simulink model "OMAP"  (R2018b)
settings: Solver=FixedStepDiscrete  StartTime=0.0  StopTime=10.0  FixedStep=0.01  RelTol=1e-3
values from neighbouring files (symbols this model uses):
  Clb_ICADirect_LaneDisp_StateFive = Simulink.Parameter    [omap_ver_442.m]
  Clb_ICADirect_LaneDisp_StateFour = Simulink.Parameter    [omap_ver_442.m]
  Clb_ICADirect_LaneDisp_StateOne = Simulink.Parameter    [omap_ver_442.m]
  Clb_ICADirect_LaneDisp_StateThree = Simulink.Parameter    [omap_ver_442.m]
  Clb_ICADirect_LaneDisp_StateTwo = Simulink.Parameter    [omap_ver_442.m]
  Clb_ICADirect_LaneDisp_StateZero = Simulink.Parameter    [omap_ver_442.m]
  Clb_ICADirect_LaneDispSW = Simulink.Parameter    [omap_ver_442.m]
  Clb_ICADirect_TrnLghtsCom_Switch = Simulink.Parameter    [omap_ver_442.m]
  Clb_ICADirect_TrnLghtsCom_Value = Simulink.Parameter    [omap_ver_442.m]
  Clb_ICADirect_TrnLghtsCrtl_Inhb = Simulink.Parameter    [omap_ver_442.m]
  OMAP_ACCAEB_EMSESC_Decel = Simulink.Parameter    [omap_ver_442.m]
  OMAP_ACCFCW_IC_Decel = Simulink.Parameter    [omap_ver_442.m]
  OMAP_clb_ACC_RVVReqType = Simulink.Parameter    [omap_ver_442.m]
  OMAP_clb_ACC_RVVReqType_Switch = Simulink.Parameter    [omap_ver_442.m]
  OMAP_clb_ACCHeadwayDisplay = Simulink.Parameter    [omap_ver_442.m]
  OMAP_clb_ACCHeadwayDisplay_Switch = Simulink.Parameter    [omap_ver_442.m]
  OMAP_clb_ACCHeadwayIcon = Simulink.Parameter    [omap_ver_442.m]
  OMAP_clb_ACCHeadwayIcon_Switch = Simulink.Parameter    [omap_ver_442.m]
  OMAP_clb_ACCMessagePrompt = Simulink.Parameter    [omap_ver_442.m]
  OMAP_clb_ACCMessagePrompt_Switch = Simulink.Parameter    [omap_ver_442.m]
  OMAP_clb_ACCRequestEPB = Simulink.Parameter    [omap_ver_442.m]
  OMAP_clb_ACCRequestEPB_Switch = Simulink.Parameter    [omap_ver_442.m]
  OMAP_clb_ACCSetSpeed = Simulink.Parameter    [omap_ver_442.m]
  OMAP_clb_ACCSetSpeed_Switch = Simulink.Parameter    [omap_ver_442.m]
  OMAP_clb_ACCSetSpeedDis = Simulink.Parameter    [omap_ver_442.m]
  OMAP_clb_ACCSetSpeedDis_Switch = Simulink.Parameter    [omap_ver_442.m]
  OMAP_clb_ACCState = Simulink.Parameter    [omap_ver_442.m]
  OMAP_clb_ACCState_Switch = Simulink.Parameter    [omap_ver_442.m]
  OMAP_clb_ACCStatusIconDis = Simulink.Parameter    [omap_ver_442.m]
  OMAP_clb_ACCStatusIconDis_Switch = Simulink.Parameter    [omap_ver_442.m]
  OMAP_clb_ACCTorqueReq = Simulink.Parameter    [omap_ver_442.m]
  OMAP_clb_ACCTorqueReq_Switch = Simulink.Parameter    [omap_ver_442.m]
  OMAP_clb_ADAS_State = Simulink.Parameter    [omap_ver_442.m]
  OMAP_clb_ADAS_State_Switch = Simulink.Parameter    [omap_ver_442.m]
  OMAP_clb_AEBAlertReq = Simulink.Parameter    [omap_ver_442.m]
  OMAP_clb_AEBAlertReq_Switch = Simulink.Parameter    [omap_ver_442.m]
  OMAP_clb_AEBBrakingProg = Simulink.Parameter    [omap_ver_442.m]
  OMAP_clb_AEBBrakingProg_Switch = Simulink.Parameter    [omap_ver_442.m]
  OMAP_clb_AEBFaultStatus = Simulink.Parameter    [omap_ver_442.m]
  OMAP_clb_AEBFaultStatus_Switch = Simulink.Parameter    [omap_ver_442.m]
  OMAP_clb_AEBMassageDisp = Simulink.Parameter    [omap_ver_442.m]
  OMAP_clb_AEBMassageDisp_Switch = Simulink.Parameter    [omap_ver_442.m]
  OMAP_clb_AEBState = Simulink.Parameter    [omap_ver_442.m]
  OMAP_clb_AEBState_Switch = Simulink.Parameter    [omap_ver_442.m]
  OMAP_clb_AEBSwitchStatus = Simulink.Parameter    [omap_ver_442.m]
  OMAP_clb_AEBSwitchStatus_Switch = Simulink.Parameter    [omap_ver_442.m]
  OMAP_clb_BrakeRequest = Simulink.Parameter    [omap_ver_442.m]
  OMAP_clb_BrakeRequest_Switch = Simulink.Parameter    [omap_ver_442.m]
  OMAP_clb_DecelerationSet = Simulink.Parameter    [omap_ver_442.m]
  OMAP_clb_DecelerationSet_Switch = Simulink.Parameter    [omap_ver_442.m]
  OMAP_clb_DecelerationType = Simulink.Parameter    [omap_ver_442.m]
  OMAP_clb_DecelerationType_Switch = Simulink.Parameter    [omap_ver_442.m]
  OMAP_clb_DeclControlReq = Simulink.Parameter    [omap_ver_442.m]
  OMAP_clb_DeclControlReq_Switch = Simulink.Parameter    [omap_ver_442.m]
  OMAP_clb_DownorUpGearMinTime = Simulink.Parameter    [omap_ver_442.m]
  OMAP_clb_DownorUpGearMinTime_Switch = Simulink.Parameter    [omap_ver_442.m]
  OMAP_clb_ELKPopupMessage = Simulink.Parameter    [omap_ver_442.m]
  OMAP_clb_ELKPopupMessage_Switch = Simulink.Parameter    [omap_ver_442.m]
  OMAP_clb_ELKSts = Simulink.Parameter    [omap_ver_442.m]
  OMAP_clb_ELKSts_Switch = Simulink.Parameter    [omap_ver_442.m]
  OMAP_clb_ESAFaultSt = Simulink.Parameter    [omap_ver_442.m]
  OMAP_clb_ESAFaultSt_Switch = Simulink.Parameter    [omap_ver_442.m]
  OMAP_clb_ESARequest = Simulink.Parameter    [omap_ver_442.m]
  OMAP_clb_ESARequest_Switch = Simulink.Parameter    [omap_ver_442.m]
  OMAP_clb_ESAState = Simulink.Parameter    [omap_ver_442.m]
  OMAP_clb_ESAState_Switch = Simulink.Parameter    [omap_ver_442.m]
  OMAP_clb_ESATorqueReq = Simulink.Parameter    [omap_ver_442.m]
  OMAP_clb_ESATorqueReq_Switch = Simulink.Parameter    [omap_ver_442.m]
  OMAP_clb_ESCDriveOff = Simulink.Parameter    [omap_ver_442.m]
  OMAP_clb_ESCDriveOff_Switch = Simulink.Parameter    [omap_ver_442.m]
  OMAP_clb_ESCHoldReq = Simulink.Parameter    [omap_ver_442.m]
  OMAP_clb_ESCHoldReq_Switch = Simulink.Parameter    [omap_ver_442.m]
  OMAP_clb_Handsoffwarning = Simulink.Parameter    [omap_ver_442.m]
  OMAP_clb_Handsoffwarning_Switch = Simulink.Parameter    [omap_ver_442.m]
  OMAP_clb_HapticAlarmReq = Simulink.Parameter    [omap_ver_442.m]
  OMAP_clb_HapticAlarmReq_Switch = Simulink.Parameter    [omap_ver_442.m]
  OMAP_clb_HMIPopupMassage = Simulink.Parameter    [omap_ver_442.m]
  OMAP_clb_HMIPopupMassage_Switch = Simulink.Parameter    [omap_ver_442.m]
  OMAP_clb_HWAActionSts = Simulink.Parameter    [omap_ver_442.m]
  OMAP_clb_HWAActionSts_Switch = Simulink.Parameter    [omap_ver_442.m]
  OMAP_clb_HWAMode = Simulink.Parameter    [omap_ver_442.m]
  OMAP_clb_HWAMode_Switch = Simulink.Parameter    [omap_ver_442.m]
  OMAP_clb_HWATurnOnIdctr = Simulink.Parameter    [omap_ver_442.m]
  OMAP_clb_HWATurnOnIdctr_Switch = Simulink.Parameter    [omap_ver_442.m]
  OMAP_clb_ICAMassageDisp = Simulink.Parameter    [omap_ver_442.m]
  OMAP_clb_ICAMassageDisp_Switch = Simulink.Parameter    [omap_ver_442.m]
  OMAP_clb_ICAStatusIcon = Simulink.Parameter    [omap_ver_442.m]
  OMAP_clb_ICAStatusIcon_Switch = Simulink.Parameter    [omap_ver_442.m]
  OMAP_clb_ISLCDriverRemind = Simulink.Parameter    [omap_ver_442.m]
  OMAP_clb_ISLCDriverRemind_Switch = Simulink.Parameter    [omap_ver_442.m]
  OMAP_clb_ISLCState = Simulink.Parameter    [omap_ver_442.m]
  OMAP_clb_ISLCState_Switch = Simulink.Parameter    [omap_ver_442.m]
  OMAP_clb_JAFaultSt = Simulink.Parameter    [omap_ver_442.m]
  OMAP_clb_JAFaultSt_Switch = Simulink.Parameter    [omap_ver_442.m]
  OMAP_clb_LCAPopupMessage = Simulink.Parameter    [omap_ver_442.m]
  OMAP_clb_LCAPopupMessage_Switch = Simulink.Parameter    [omap_ver_442.m]
  OMAP_clb_LCAStatusDisplay = Simulink.Parameter    [omap_ver_442.m]
  OMAP_clb_LCAStatusDisplay_Switch = Simulink.Parameter    [omap_ver_442.m]
  OMAP_clb_LDWStatusDisplay = Simulink.Parameter    [omap_ver_442.m]
  OMAP_clb_LDWStatusDisplay_Switch = Simulink.Parameter    [omap_ver_442.m]
  OMAP_clb_LDWWarningSt = Simulink.Parameter    [omap_ver_442.m]
  OMAP_clb_LDWWarningSt_Switch = Simulink.Parameter    [omap_ver_442.m]
  OMAP_clb_LightControlValid = Simulink.Parameter    [omap_ver_442.m]
  OMAP_clb_LightControlValid_Switch = Simulink.Parameter    [omap_ver_442.m]
  OMAP_clb_LKAActivation = Simulink.Parameter    [omap_ver_442.m]
  OMAP_clb_LKAActivation_Switch = Simulink.Parameter    [omap_ver_442.m]
  OMAP_clb_LKAAngleReq = Simulink.Parameter    [omap_ver_442.m]
  OMAP_clb_LKAAngleReq_Switch = Simulink.Parameter    [omap_ver_442.m]
  OMAP_clb_LKAMode = Simulink.Parameter    [omap_ver_442.m]
  OMAP_clb_LKAMode_Switch = Simulink.Parameter    [omap_ver_442.m]
  OMAP_clb_LKAorELK_CoolTime = Simulink.Parameter    [omap_ver_442.m]
  OMAP_clb_LKAState = Simulink.Parameter    [omap_ver_442.m]
  OMAP_clb_LKAState_Switch = Simulink.Parameter    [omap_ver_442.m]
  OMAP_clb_LKAStatusDisplay = Simulink.Parameter    [omap_ver_442.m]
  OMAP_clb_LKAStatusDisplay_Switch = Simulink.Parameter    [omap_ver_442.m]
  OMAP_clb_LKASwitchState = Simulink.Parameter    [omap_ver_442.m]
  OMAP_clb_LKASwitchState_Switch = Simulink.Parameter    [omap_ver_442.m]
  OMAP_clb_LKATorqFactReq = Simulink.Parameter    [omap_ver_442.m]
  OMAP_clb_LKATorqFactReq_Switch = Simulink.Parameter    [omap_ver_442.m]
  OMAP_clb_PrefillRequest = Simulink.Parameter    [omap_ver_442.m]
  ... (+36 more)
libraries: simulink x184, canmsglib x2
(part 11 of 14)

== system OMAP/Runnable_OMAP_10ms_sys/OMAP_Module/ACCS_Direct/ACCS_Define/Human_Machine_Interface(ACC_HMI)/Text_PopUp/ACC_Canceled ==
  In1 : Inport
  Chart : Stateflow chart  TreatAsAtomicUnit=on
  Compare To Constant1 : simulink/Logic and Bit Operations/Compare To Constant  relop===  const=2  OutDataTypeStr=boolean
  Compare To Constant2 : simulink/Logic and Bit Operations/Compare To Constant  relop===  const=3  OutDataTypeStr=boolean
  Compare To Constant23 : simulink/Logic and Bit Operations/Compare To Constant  relop===  const=4  OutDataTypeStr=boolean
  Compare To Constant3 : simulink/Logic and Bit Operations/Compare To Constant  relop===  const=7  OutDataTypeStr=boolean
  Compare To Constant4 : simulink/Logic and Bit Operations/Compare To Constant  relop===  const=6  OutDataTypeStr=boolean
  Compare To Constant5 : simulink/Logic and Bit Operations/Compare To Constant  relop===  const=2  OutDataTypeStr=boolean
  Compare To Constant6 : simulink/Logic and Bit Operations/Compare To Constant  relop===  const=3  OutDataTypeStr=boolean
  Compare To Constant7 : simulink/Logic and Bit Operations/Compare To Constant  relop===  const=5  OutDataTypeStr=boolean
  Logical Operator1 : Logic  Operator=OR  Inputs=3  AllPortsSameDT=off  OutDataTypeStr=boolean
  Logical Operator16 : Logic  AllPortsSameDT=off  OutDataTypeStr=boolean
  Logical Operator2 : Logic  Operator=OR  AllPortsSameDT=off  OutDataTypeStr=boolean
  Logical Operator3 : Logic  Operator=OR  AllPortsSameDT=off  OutDataTypeStr=boolean
  Logical Operator4 : Logic  AllPortsSameDT=off  OutDataTypeStr=boolean
  Logical Operator5 : Logic  Operator=OR  AllPortsSameDT=off  OutDataTypeStr=boolean
  Unit Delay1 : UnitDelay  SampleTime=-1
  Unit Delay5 : UnitDelay  SampleTime=-1
  Out1 : Outport
  wires:
  Compare To Constant1/1 -> Logical Operator1/1
  Compare To Constant23/1 -> Logical Operator16/1
  Logical Operator16/1 -> Logical Operator2/1
  Chart/1(Value) -> Out1/1
  Unit Delay5/1 -> Compare To Constant23/1
  Compare To Constant2/1 -> Logical Operator1/2
  Compare To Constant3/1 -> Logical Operator1/3
  Logical Operator1/1 -> Logical Operator16/2
  Compare To Constant5/1 -> Logical Operator3/1
  Compare To Constant7/1 -> Logical Operator5/1
  In1/1 -> Compare To Constant6/1, Compare To Constant5/1, Unit Delay1/1, Compare To Constant3/1, Compare To Constant2/1, Compare To Constant1/1, Unit Delay5/1
  Unit Delay1/1 -> Compare To Constant4/1, Compare To Constant7/1
  Compare To Constant6/1 -> Logical Operator3/2
  Logical Operator3/1 -> Logical Operator4/2
  Logical Operator4/1 -> Logical Operator2/2
  Logical Operator2/1 -> Chart/1(data)
  Compare To Constant4/1 -> Logical Operator5/2
  Logical Operator5/1 -> Logical Operator4/1

== system OMAP/Runnable_OMAP_10ms_sys/OMAP_Module/ACCS_Direct/ACCS_Define/Human_Machine_Interface(ACC_HMI)/Text_PopUp/ACC_Fault ==
  In1 : Inport
  Chart : Stateflow chart  TreatAsAtomicUnit=on
  Compare To Constant1 : simulink/Logic and Bit Operations/Compare To Constant  relop=~=  const=15  OutDataTypeStr=boolean
  Compare To Constant15 : simulink/Logic and Bit Operations/Compare To Constant  relop===  const=15  OutDataTypeStr=boolean
  Logical Operator : Logic  AllPortsSameDT=off  OutDataTypeStr=boolean
  Unit Delay : UnitDelay  SampleTime=-1
  Out1 : Outport
  wires:
  Logical Operator/1 -> Chart/1(data)
  In1/1 -> Compare To Constant15/1, Unit Delay/1
  Compare To Constant1/1 -> Logical Operator/1
  Compare To Constant15/1 -> Logical Operator/2
  Unit Delay/1 -> Compare To Constant1/1
  Chart/1(Value) -> Out1/1

== system OMAP/Runnable_OMAP_10ms_sys/OMAP_Module/ACCS_Direct/ACCS_Define/Human_Machine_Interface(ACC_HMI)/Text_PopUp/ACC_OFF ==
  In1 : Inport
  In2 : Inport  Port=2
  Chart : Stateflow chart  TreatAsAtomicUnit=on
  Compare To Constant1 : simulink/Logic and Bit Operations/Compare To Constant  relop===  const=1  OutDataTypeStr=boolean
  Compare To Constant10 : simulink/Logic and Bit Operations/Compare To Constant  relop===  const=8  OutDataTypeStr=boolean
  Compare To Constant2 : simulink/Logic and Bit Operations/Compare To Constant  relop=~=  const=0  OutDataTypeStr=boolean
  Compare To Constant3 : simulink/Logic and Bit Operations/Compare To Constant  relop=~=  const=15  OutDataTypeStr=boolean
  Compare To Constant4 : simulink/Logic and Bit Operations/Compare To Constant  relop=~=  const=1  OutDataTypeStr=boolean
  Compare To Constant5 : simulink/Logic and Bit Operations/Compare To Constant  relop=~=  const=8  OutDataTypeStr=boolean
  Compare To Constant6 : simulink/Logic and Bit Operations/Compare To Constant  relop===  const=0  OutDataTypeStr=boolean
  Compare To Constant7 : simulink/Logic and Bit Operations/Compare To Constant  relop===  const=1  OutDataTypeStr=boolean
  Compare To Constant8 : simulink/Logic and Bit Operations/Compare To Constant  relop===  const=4  OutDataTypeStr=boolean
  Logical Operator1 : Logic  Inputs=4  AllPortsSameDT=off  OutDataTypeStr=boolean
  Logical Operator2 : Logic  AllPortsSameDT=off  OutDataTypeStr=boolean
  Logical Operator3 : Logic  AllPortsSameDT=off  OutDataTypeStr=boolean
  Logical Operator4 : Logic  Operator=OR  AllPortsSameDT=off  OutDataTypeStr=boolean
  Logical Operator5 : Logic  AllPortsSameDT=off  OutDataTypeStr=boolean
  Unit Delay1 : UnitDelay  SampleTime=-1
  Unit Delay2 : UnitDelay  SampleTime=-1
  Unit Delay6 : UnitDelay  SampleTime=-1
  Out1 : Outport
  wires:
  Unit Delay6/1 -> Compare To Constant8/1
  Logical Operator3/1 -> Logical Operator4/1
  Compare To Constant10/1 -> Logical Operator3/2
  Compare To Constant8/1 -> Logical Operator3/1
  Chart/1(Value) -> Out1/1
  Unit Delay1/1 -> Compare To Constant5/1, Compare To Constant4/1, Compare To Constant3/1, Compare To Constant2/1
  Compare To Constant1/1 -> Logical Operator2/2
  Compare To Constant2/1 -> Logical Operator1/1
  In1/1 -> Unit Delay1/1, Compare To Constant1/1, Compare To Constant10/1, Unit Delay6/1
  Compare To Constant3/1 -> Logical Operator1/2
  Compare To Constant4/1 -> Logical Operator1/3
  Compare To Constant5/1 -> Logical Operator1/4
  Logical Operator1/1 -> Logical Operator2/1
  Logical Operator2/1 -> Logical Operator4/2
  Logical Operator4/1 -> Chart/1(data)
  In2/1 -> Unit Delay2/1, Compare To Constant6/1
  Compare To Constant7/1 -> Logical Operator5/1
  Compare To Constant6/1 -> Logical Operator5/2
  Unit Delay2/1 -> Compare To Constant7/1
  Logical Operator5/1 -> Chart/2(data1)

== system OMAP/Runnable_OMAP_10ms_sys/OMAP_Module/ACCS_Direct/ACCS_Define/Human_Machine_Interface(ACC_HMI)/Text_PopUp/ACC_ON ==
  In1 : Inport
  In2 : Inport  Port=2
  ACCICA_Flag : Inport  Port=3
  Chart : Stateflow chart  TreatAsAtomicUnit=on
  Compare To Constant{1..2,6,9} (4 alike) : simulink/Logic and Bit Operations/Compare To Constant  relop===  const=1  OutDataTypeStr=boolean
  Compare To Constant10 : simulink/Logic and Bit Operations/Compare To Constant  relop=~=  const=1  OutDataTypeStr=boolean
  Compare To Constant11 : simulink/Logic and Bit Operations/Compare To Constant  relop=~=  const=15  OutDataTypeStr=boolean
  Compare To Constant14 : simulink/Logic and Bit Operations/Compare To Constant  relop===  const=3  OutDataTypeStr=boolean
  Compare To Constant3 : simulink/Logic and Bit Operations/Compare To Constant  relop===  const=2  OutDataTypeStr=boolean
  Compare To Constant4 : simulink/Logic and Bit Operations/Compare To Constant  relop=~=  const=1  OutDataTypeStr=boolean
  Compare To Constant5 : simulink/Logic and Bit Operations/Compare To Constant  relop=~=  const=0  OutDataTypeStr=boolean
  Compare To Constant7 : simulink/Logic and Bit Operations/Compare To Constant  relop===  const=0  OutDataTypeStr=boolean
  Compare To Constant8 : simulink/Logic and Bit Operations/Compare To Constant  relop===  const=0  OutDataTypeStr=boolean
  Logical Operator : Logic  Inputs=3  AllPortsSameDT=off  OutDataTypeStr=boolean
  Logical Operator1 : Logic  AllPortsSameDT=off  OutDataTypeStr=boolean
  Logical Operator2 : Logic  AllPortsSameDT=off  OutDataTypeStr=boolean
  Logical Operator3 : Logic  AllPortsSameDT=off  OutDataTypeStr=boolean
  Logical Operator4 : Logic  Operator=OR  AllPortsSameDT=off  OutDataTypeStr=boolean
  Logical Operator5 : Logic  Inputs=3  AllPortsSameDT=off  OutDataTypeStr=boolean
  Logical Operator9 : Logic  Operator=OR  AllPortsSameDT=off  OutDataTypeStr=boolean
  Unit Delay : UnitDelay  SampleTime=-1
  Unit Delay1 : UnitDelay  SampleTime=-1
  Unit Delay2 : UnitDelay  SampleTime=-1
  Out1 : Outport
  wires:
  Compare To Constant14/1 -> Logical Operator9/2
  Compare To Constant1/1 -> Logical Operator/1
  Logical Operator/1 -> Chart/1(data)
  Logical Operator9/1 -> Logical Operator/2
  Unit Delay/1 -> Compare To Constant1/1
  Compare To Constant3/1 -> Logical Operator9/1
  Chart/1(Value) -> Out1/1
  In2/1 -> Compare To Constant4/1, Unit Delay1/1
  Unit Delay1/1 -> Compare To Constant2/1
  Compare To Constant2/1 -> Logical Operator1/1
  Compare To Constant4/1 -> Logical Operator1/2
  Logical Operator4/1 -> Chart/2(data1)
  In1/1 -> Compare To Constant11/1, Compare To Constant10/1, Compare To Constant5/1, Compare To Constant14/1, Compare To Constant3/1, Unit Delay/1
  Logical Operator5/1 -> Logical Operator2/2
  ACCICA_Flag/1 -> Compare To Constant8/1, Compare To Constant9/1, Compare To Constant7/1, Unit Delay2/1
  Unit Delay2/1 -> Compare To Constant6/1
  Compare To Constant6/1 -> Logical Operator3/1
  Compare To Constant7/1 -> Logical Operator3/2
  Logical Operator3/1 -> Logical Operator2/1
  Logical Operator2/1 -> Chart/3(data2)
  Compare To Constant8/1 -> Logical Operator/3
  Logical Operator1/1 -> Logical Operator4/2
  Compare To Constant9/1 -> Logical Operator4/1
  Compare To Constant5/1 -> Logical Operator5/1
  Compare To Constant10/1 -> Logical Operator5/2
  Compare To Constant11/1 -> Logical Operator5/3

== system OMAP/Runnable_OMAP_10ms_sys/OMAP_Module/ACCS_Direct/ACCS_Define/Human_Machine_Interface(ACC_HMI)/Text_PopUp/ACC_go_request ==
  In1 : Inport
  Compare To Constant1 : simulink/Logic and Bit Operations/Compare To Constant  relop===  const=1  OutDataTypeStr=boolean
  <GoRequest> : Outport
  wires:
  In1/1 -> Compare To Constant1/1
  Compare To Constant1/1 -> <GoRequest>/1

== system OMAP/Runnable_OMAP_10ms_sys/OMAP_Module/ACCS_Direct/ACCS_Define/Human_Machine_Interface(ACC_HMI)/Text_PopUp/Please_Take_Over_the_Car ==
  In1 : Inport
  Chart1 : Stateflow chart  TreatAsAtomicUnit=on
  Compare To Constant1 : simulink/Logic and Bit Operations/Compare To Constant  relop===  const=6  OutDataTypeStr=boolean
  Compare To Constant18 : simulink/Logic and Bit Operations/Compare To Constant  relop===  const=6  OutDataTypeStr=boolean
  Compare To Constant19 : simulink/Logic and Bit Operations/Compare To Constant  relop===  const=4  OutDataTypeStr=boolean
  Compare To Constant2 : simulink/Logic and Bit Operations/Compare To Constant  relop=~=  const=6  OutDataTypeStr=boolean
  Logical Operator1 : Logic  AllPortsSameDT=off  OutDataTypeStr=boolean
  Logical Operator7 : Logic  AllPortsSameDT=off  OutDataTypeStr=boolean
  Unit Delay1 : UnitDelay  SampleTime=-1
  Unit Delay2 : UnitDelay  SampleTime=-1
  Out1 : Outport
  wires:
  Logical Operator7/1 -> Chart1/1(IN)
  Compare To Constant18/1 -> Logical Operator7/2
  Unit Delay2/1 -> Compare To Constant19/1
  Compare To Constant19/1 -> Logical Operator7/1
  Chart1/1(Value) -> Out1/1
  Unit Delay1/1 -> Compare To Constant1/1
  Compare To Constant1/1 -> Logical Operator1/1
  Compare To Constant2/1 -> Logical Operator1/2
  Logical Operator1/1 -> Chart1/2(OUT)
  In1/1 -> Unit Delay1/1, Compare To Constant2/1, Compare To Constant18/1, Unit Delay2/1

== system OMAP/Runnable_OMAP_10ms_sys/OMAP_Module/ACCS_Direct/ACCS_Define/Human_Machine_Interface(ACC_HMI)/Text_PopUp/Please_Take_Over_the_Car_immediataly ==
  ESC_DecTar : Inport
  BRAKE_RELEASED_FAILSAFE1 : Constant  Value=0  OutDataTypeStr=boolean
  Chart1 : Stateflow chart  TreatAsAtomicUnit=on
  Out1 : Outport
  wires:
  Chart1/1(Value) -> Out1/1
  ESC_DecTar/1 -> Chart1/1(ESC_DecTar)
  BRAKE_RELEASED_FAILSAFE1/1 -> Chart1/2(BRAKE_RELEASED_FAILSAFE)

== system OMAP/Runnable_OMAP_10ms_sys/OMAP_Module/ICA_Direct_G59/ICA_Define/Subsystem1/Dspl/DsplPrcs ==
  note: 0是运动，1是静止
  note: 0是脱手，1是不脱手
  DsplPrcs_stStWhlHld : Inport
  DsplPrcs_stTkOvStChk : Inport  Port=2
  DsplPrcs_facmL0Ql : Inport  Port=3
  DsplPrcs_facmR0Ql : Inport  Port=4
  DsplPrcs_facmL0Type : Inport  Port=5
  DsplPrcs_facmR0Type : Inport  Port=6
  DsplPrcs_stTHState : Inport  Port=7
  DsplPrcs_bsFromFMCMsg : Inport  Port=8
  DsplPrcs_stTHFKeyState : Inport  Port=9
  DsplPrcs_stVehSty : Inport  Port=10
  DsplPrcs_tfAddVocCmd : Inport  Port=11
  DsplPrcs_stSWALimFlg : Inport  Port=12
  DsplPrcs_dDgrdIconWarnflag : Inport  Port=13
  DsplPrcs_stturn_lightState : Inport  Port=14
  DsplPrcs_stTLC_ALCmodeSW : Inport  Port=15
  DsplPrcs_stLC_SpdCndtFlg : Inport  Port=16
  DsplPrcs_dHndOffTxtWarnnum : Inport  Port=17
  DsplPrcs_dDgrdVocWarnDurnum : Inport  Port=18
  DsplPrcs_dHndOffVocWarnnum : Inport  Port=19
  DsplPrcs_dTxtLimnum : Inport  Port=20
  DsplPrcs_dDgrdIconWarnHiDurnum : Inport  Port=21
  DsplPrcs_dDgrdIconWarnLoDurnum : Inport  Port=22
  DsplPrcs_tiSWALimFlgDetnum : Inport  Port=23
  Bus Creator1 : BusCreator  Inputs=4
  Bus Selector : BusSelector  OutputSignals=stLaneDspl,stL0DispType,stR0DispType
  Bus Selector1 : BusSelector  OutputSignals=ACC_State
  Bus Selector2 : BusSelector  OutputSignals=Icon_stICAIcon,Icon_stHWAmode
  Data Type Conversion1 : DataTypeConversion  OutDataTypeStr=uint16
  Icon : Subsystem
  Lane : Subsystem
  Txt : Subsystem
  Voc : Subsystem
  DsplPrcs_stTxtDspl : Outport
  DsplPrcs_stICAIcon : Outport  Port=2
  DsplPrcs_stLaneDspl : Outport  Port=3
  DsplPrcs_stL0DispType : Outport  Port=4
  DsplPrcs_stR0DispType : Outport  Port=5
  DsplPrcs_stVocDspl : Outport  Port=6
  DsplPrcs_stHWAmode : Outport  Port=7
  DsplPrcs_bsMon : Outport  Port=8
  wires:
  DsplPrcs_stTHFKeyState/1 -> Txt/4(Txt_stTHFKeyState)
  Txt/1(Txt_stTxtDspl) -> DsplPrcs_stTxtDspl/1
  DsplPrcs_stTHState/1 -> Voc/2(Voc_stTHState), Lane/1(Lane_stTHState), Icon/1(Icon_stTHState), Txt/6(Txt_stTHState)
  Icon/1(Icon_stIconDspl) -> Bus Creator1/2, Bus Selector2/1  "stIconDspl"
  Lane/1(Lane_stLaneDspl) -> Bus Selector/1, Bus Creator1/3  "Vehicle_Lane_Display"
  Txt/2(Txt_bsMon) -> Bus Creator1/1  "ICA_HMI_Txt_Mon"
  Bus Creator1/1 -> DsplPrcs_bsMon/1
  DsplPrcs_stStWhlHld/1 -> Txt/1(Txt_stStWhlHld), Voc/1(Voc_stStWhlHld)
  DsplPrcs_dHndOffTxtWarnnum/1 -> Txt/5(Txt_dHndOffTxtWarnnum)
  Voc/1(Voc_stVocDspl) -> DsplPrcs_stVocDspl/1, Bus Creator1/4  "Hands_off_warning"
  DsplPrcs_dHndOffVocWarnnum/1 -> Voc/4(Voc_dHndOffVocWarnnum)
  DsplPrcs_dDgrdVocWarnDurnum/1 -> Voc/3(Voc_dDgrdVocWarnDurnum)
  DsplPrcs_bsFromFMCMsg/1 -> Bus Selector1/1, Txt/3(Txt_bsFromFMCMsg)
  Data Type Conversion1/1 -> Icon/2(Icon_stACCState)
  Bus Selector1/1 -> Data Type Conversion1/1  "<ACC_State>"
  DsplPrcs_dTxtLimnum/1 -> Txt/7(Txt_dTxtLimnum)
  DsplPrcs_facmL0Ql/1 -> Lane/3(Lane_facmL0Ql)
  DsplPrcs_facmR0Ql/1 -> Lane/4(Lane_facmR0Ql)
  DsplPrcs_stVehSty/1 -> Txt/2(Txt_stVehSty), Lane/2(Lane_stVehSty), Voc/5(Voc_stVehSty)
  DsplPrcs_tfAddVocCmd/1 -> Txt/11(Txt_tfAddVocCmd)
  DsplPrcs_dDgrdIconWarnHiDurnum/1 -> Icon/3(Icon_dDgrdIconWarnHiDurnum)
  DsplPrcs_dDgrdIconWarnLoDurnum/1 -> Icon/4(Icon_dDgrdIconWarnLoDurnum)
  DsplPrcs_dDgrdIconWarnflag/1 -> Icon/5(Icon_dDgrdIconWarnflag)
  DsplPrcs_stSWALimFlg/1 -> Txt/8(Txt_stSWALimFlg)
  DsplPrcs_tiSWALimFlgDetnum/1 -> Txt/9(Txt_tiSWALimFlgDetnum)
  DsplPrcs_facmL0Type/1 -> Lane/5(Lane_facmL0Type)
  DsplPrcs_facmR0Type/1 -> Lane/6(Lane_facmR0Type)
  Bus Selector/1 -> DsplPrcs_stLaneDspl/1  "<stLaneDspl>"
  Bus Selector/2 -> DsplPrcs_stL0DispType/1  "<stL0DispType>"
  Bus Selector/3 -> DsplPrcs_stR0DispType/1  "<stR0DispType>"
  DsplPrcs_stturn_lightState/1 -> Lane/7(Lane_stturn_lightState)
  DsplPrcs_stTLC_ALCmodeSW/1 -> Lane/8(Lane_stTLC_ALCmodeSW)
  DsplPrcs_stTkOvStChk/1 -> Txt/10(Txt_stTkOvStChk), Icon/6(Icon_stTLC_ALCmodeSW), Lane/9(Lane_stTkOvStChk)
  DsplPrcs_stLC_SpdCndtFlg/1 -> Icon/7(Icon_stLC_SpdCndtFlg)
  Bus Selector2/2 -> DsplPrcs_stHWAmode/1  "<Icon_stHWAmode>"
  Bus Selector2/1 -> DsplPrcs_stICAIcon/1  "<Icon_stICAIcon>"

== system OMAP/Runnable_OMAP_10ms_sys/OMAP_Module/ICA_Direct_G59/ICA_Define/Subsystem1/Dspl/TimePrcs ==
  note: 降级图标闪烁的单次点亮时间，1.3s
  note: 文字提示的最长显示时间，3s
  note: 方向盘转角限幅报警的时间阈值
  note: 功能降级声音提示时长，0.5s
  note: 降级图标闪烁的单次熄灭时间，0.2s
  TimePrcs_tiHndOffTxtWarnT_C : Inport
  TimePrcs_tiDgrdVocWarnDurT_C : Inport  Port=2
  TimePrcs_tiHndOffVocWarnT_C : Inport  Port=3
  TimePrcs_tiTxtLimT_C : Inport  Port=4
  TimePrcs_tiDgrdIconWarnHiDurT_C : Inport  Port=5
  TimePrcs_tiDgrdIconWarnLoDurT_C : Inport  Port=6
  TimePrcs_tiSWALimFlgDetT_C : Inport  Port=7
  TimePrcs_tiCalcPer_C : Inport  Port=8
  Divide{,1..6} (7 alike) : Product  Inputs=*/  OutDataTypeStr=uint16
  Switch : Switch  Criteria=u2 ~= 0  OutDataTypeStr=single
  constant : Constant  Value=0.01  OutDataTypeStr=single
  TimePrcs_dHndOffTxtWarnnum : Outport
  TimePrcs_dDgrdVocWarnDurnum : Outport  Port=2
  TimePrcs_dHndOffVocWarnnum : Outport  Port=3
  TimePrcs_dTxtLimnum : Outport  Port=4
  TimePrcs_dDgrdIconWarnHiDurnum : Outport  Port=5
  TimePrcs_dDgrdIconWarnLoDurnum : Outport  Port=6
  TimePrcs_tiSWALimFlgDetnum : Outport  Port=7
  wires:
  Divide/1 -> TimePrcs_dHndOffTxtWarnnum/1
  TimePrcs_tiCalcPer_C/1 -> Switch/1, Switch/2
  constant/1 -> Switch/3
  TimePrcs_tiHndOffTxtWarnT_C/1 -> Divide/1
  Switch/1 -> Divide5/2, Divide4/2, Divide3/2, Divide2/2, Divide1/2, Divide/2, Divide6/2
  TimePrcs_tiDgrdVocWarnDurT_C/1 -> Divide1/1
  TimePrcs_tiHndOffVocWarnT_C/1 -> Divide2/1
  TimePrcs_tiTxtLimT_C/1 -> Divide3/1
  Divide1/1 -> TimePrcs_dDgrdVocWarnDurnum/1
  Divide2/1 -> TimePrcs_dHndOffVocWarnnum/1
  Divide3/1 -> TimePrcs_dTxtLimnum/1
  TimePrcs_tiDgrdIconWarnHiDurT_C/1 -> Divide4/1
  Divide4/1 -> TimePrcs_dDgrdIconWarnHiDurnum/1
  TimePrcs_tiDgrdIconWarnLoDurT_C/1 -> Divide5/1
  Divide5/1 -> TimePrcs_dDgrdIconWarnLoDurnum/1
  Divide6/1 -> TimePrcs_tiSWALimFlgDetnum/1
  TimePrcs_tiSWALimFlgDetT_C/1 -> Divide6/1

== system OMAP/Runnable_OMAP_10ms_sys/OMAP_Module/ICA_Direct_G59/ICA_Define/Subsystem1/Subsystem/Subsystem ==
  HiDurnum : Inport
  LoDurnum : Inport  Port=2
  Add : Sum
  Constant1 : Constant  Value=0  OutDataTypeStr=uint16
  Constant8 : Constant  OutDataTypeStr=uint16
  Count : Terminator
  Relational Operator1 : RelationalOperator  Operator=<=  OutDataTypeStr=boolean  RndMeth=Nearest
  Relational Operator2 : RelationalOperator  Operator=<=  OutDataTypeStr=boolean  RndMeth=Nearest
  Sum : Sum  OutDataTypeStr=Inherit: Inherit via back propagation  InputSameDT=on
  Unit Delay1 : UnitDelay  SampleTime=-1
  Unit Delay2 : UnitDelay  SampleTime=-1
  reset switch1 : Switch  Criteria=u2 ~= 0  Threshold=1  OutDataTypeStr=Inherit: Inherit via back propagation  InputSameDT=on
  Signal : Outport
  wires:
  Unit Delay2/1 -> Sum/2
  HiDurnum/1 -> Relational Operator2/2, Add/1
  Unit Delay1/1 -> [reset]
  Add/1 -> Relational Operator1/1
  [reset] -> reset switch1/2
  Constant8/1 -> Sum/1
  Relational Operator1/1 -> Unit Delay1/1
  reset switch1/1 -> Count/1, Relational Operator2/1, Relational Operator1/2, Unit Delay2/1
  Constant1/1 -> reset switch1/1
  LoDurnum/1 -> Add/2
  Relational Operator2/1 -> Signal/1
  Sum/1 -> reset switch1/3

== system OMAP/Runnable_OMAP_10ms_sys/OMAP_Module/Subsystem/EPS_Default_Arbitration/LKA_arb_ELK/Subsystem/Subsystem1 ==
  In1 : Inport
  In2 : Inport  Port=2
  Detect Fall Nonpositive : simulink/Logic and Bit Operations/Detect Fall Nonpositive  vinit=0  OutDataTypeStr=boolean
      settings: SourceProductName=Simulink  SourceProductBaseCode=SL
  Detect Rise Positive : simulink/Logic and Bit Operations/Detect Rise Positive  vinit=0  OutDataTypeStr=boolean
  If : If  NumInputs=2  IfExpression=u1  ElseIfExpressions=u2
  If Action Subsystem : Subsystem  TreatAsAtomicUnit=on
  If Action Subsystem1 : Subsystem  TreatAsAtomicUnit=on
  If Action Subsystem2 : Subsystem  TreatAsAtomicUnit=on
  Memory : Memory  InheritSampleTime=on
  Merge : Merge  Inputs=3
  Subsystem2 : Subsystem
  Out1 : Outport
  wires:
  Memory/1 -> If Action Subsystem1/1(In1)
  If Action Subsystem2/1(Out1) -> Merge/2
  If/2 -> If Action Subsystem2/Action
  Detect Rise Positive/1 -> If/2
  If/3 -> If Action Subsystem1/Action
  In1/1 -> Detect Fall Nonpositive/1, Detect Rise Positive/1
  If Action Subsystem1/1(Out1) -> Merge/3
  If/1 -> If Action Subsystem/Action
  Detect Fall Nonpositive/1 -> If/1
  Subsystem2/1(Out1) -> Memory/1, Out1/1
  In2/1 -> Subsystem2/1(In1)
  Merge/1 -> Subsystem2/Enable
  If Action Subsystem/1(Out1) -> Merge/1

== system OMAP/Runnable_OMAP_10ms_sys/OMAP_Module/Subsystem/EPS_Default_Arbitration/LKA_arb_ELK/Subsystem/Subsystem2 ==
  In1 : Inport
  In2 : Inport  Port=2
  Detect Fall Nonpositive : simulink/Logic and Bit Operations/Detect Fall Nonpositive  vinit=0  OutDataTypeStr=boolean
      settings: SourceProductName=Simulink  SourceProductBaseCode=SL
  Detect Rise Positive : simulink/Logic and Bit Operations/Detect Rise Positive  vinit=0  OutDataTypeStr=boolean
  If : If  NumInputs=2  IfExpression=u1  ElseIfExpressions=u2
  If Action Subsystem : Subsystem  TreatAsAtomicUnit=on
  If Action Subsystem1 : Subsystem  TreatAsAtomicUnit=on
  If Action Subsystem2 : Subsystem  TreatAsAtomicUnit=on
  Memory : Memory  InheritSampleTime=on
  Merge : Merge  Inputs=3
  Subsystem2 : Subsystem
  Out1 : Outport
  wires:
  If Action Subsystem/1(Out1) -> Merge/1
  Merge/1 -> Subsystem2/Enable
  In2/1 -> Subsystem2/1(In1)
  Subsystem2/1(Out1) -> Out1/1, Memory/1
  Detect Fall Nonpositive/1 -> If/1
  If/1 -> If Action Subsystem/Action
  If Action Subsystem1/1(Out1) -> Merge/3
  In1/1 -> Detect Rise Positive/1, Detect Fall Nonpositive/1
  If/3 -> If Action Subsystem1/Action
  Detect Rise Positive/1 -> If/2
  If/2 -> If Action Subsystem2/Action
  If Action Subsystem2/1(Out1) -> Merge/2
  Memory/1 -> If Action Subsystem1/1(In1)

== system OMAP/Runnable_OMAP_10ms_sys/OMAP_Module/Subsystem/EPS_Default_Arbitration/LKA_arb_ELK/Subsystem2/Subsystem1 ==
  LKA_State : Inport
  ELK_State : Inport  Port=2
  AND{,1..3} (4 alike) : Logic  AllPortsSameDT=off  OutDataTypeStr=boolean
  Compare To Constant{,2,4,6} (4 alike) : simulink/Logic and Bit Operations/Compare To Constant  relop===  const=uint8(4)  OutDataTypeStr=boolean
  Compare To Constant{1,3,5,7} (4 alike) : simulink/Logic and Bit Operations/Compare To Constant  relop=~=  const=uint8(4)  OutDataTypeStr=boolean
  Unit Delay : UnitDelay  InitialCondition=uint8(0)  SampleTime=-1
  Unit Delay1 : UnitDelay  InitialCondition=uint8(0)  SampleTime=-1
  LKA_Up : Outport
  LKA_Down : Outport  Port=2
  LKA_Active : Outport  Port=3
  ELK_Up : Outport  Port=4
  ELK_Down : Outport  Port=5
  ELK_Active : Outport  Port=6
  wires:
  LKA_State/1 -> Compare To Constant/1, Unit Delay/1, Compare To Constant3/1
  Unit Delay/1 -> Compare To Constant2/1, Compare To Constant1/1
  Compare To Constant1/1 -> AND/1
  Compare To Constant/1 -> LKA_Active/1, AND/2
  AND/1 -> LKA_Up/1  "LKA_Up"
  Compare To Constant2/1 -> AND1/1
  Compare To Constant3/1 -> AND1/2
  AND1/1 -> LKA_Down/1  "LKA_Down"
  Compare To Constant4/1 -> ELK_Active/1, AND2/2
  Compare To Constant6/1 -> AND3/1
  AND3/1 -> ELK_Down/1  "ELK_Down"
  Compare To Constant5/1 -> AND2/1
  ELK_State/1 -> Compare To Constant4/1, Unit Delay1/1, Compare To Constant7/1
  Unit Delay1/1 -> Compare To Constant6/1, Compare To Constant5/1
  AND2/1 -> ELK_Up/1  "ELK_Up"
  Compare To Constant7/1 -> AND3/2

== system OMAP/Runnable_OMAP_10ms_sys/OMAP_Module/Subsystem/ESC_Arbitration/ACC//ICA_arb_AEB//JA/AEB_arb_JA/AEB//JA_arb_ELK ==
  Input_ELKS : Inport
  AEB_Alert : Inport  Port=2
  JA_Alert : Inport  Port=3
  AEB+JA_Haptic : Inport  Port=4
  Bus Selector1 : BusSelector  OutputSignals=ELKSve_y_ELK_HapticAlarmReq_convert
  Compare To Constant1 : simulink/Logic and Bit Operations/Compare To Constant  relop=~=  const=0  OutDataTypeStr=boolean
  Compare To Constant4 : simulink/Logic and Bit Operations/Compare To Constant  relop=~=  const=0  OutDataTypeStr=boolean
  Index Vector1 : MultiPortSwitch  DataPortOrder=Zero-based contiguous  Inputs=2  zeroidx=on  OutDataTypeStr=uint8
  Logical Operator1 : Logic  Operator=OR  AllPortsSameDT=off  OutDataTypeStr=boolean
  Out1 : Outport
  wires:
  Input_ELKS/1 -> Bus Selector1/1
  Index Vector1/1 -> Out1/1
  Logical Operator1/1 -> Index Vector1/1
  Bus Selector1/1 -> Index Vector1/2  "<ELKSve_y_ELK_HapticAlarmReq_convert>"
  AEB+JA_Haptic/1 -> Index Vector1/3
  JA_Alert/1 -> Compare To Constant4/1
  Compare To Constant1/1 -> Logical Operator1/1
  AEB_Alert/1 -> Compare To Constant1/1
  Compare To Constant4/1 -> Logical Operator1/2

== system OMAP/Runnable_OMAP_10ms_sys/OMAP_Module/Subsystem/ESC_Arbitration/ACC//ICA_arb_AEB//JA/AEB_arb_JA/AEB_arb_JA_STATUS ==
  <JABSve_d_DbFunFARCSta_convert> : Inport
  <JABSve_d_DbJACWStatus_convert> : Inport  Port=2
  <AEBSve_d_FCWStatus_convert> : Inport  Port=3
  <AEBSve_d_functionFARCState_convert> : Inport  Port=4
  If : If  NumInputs=2  IfExpression=(u1==7|u2==7)  ElseIfExpressions=(u1==3&u2==3),(u1==3&u2==5),(u1==3&u2==6)
  If Action Subsystem : Subsystem  TreatAsAtomicUnit=on
  If Action Subsystem1 : Subsystem  TreatAsAtomicUnit=on
  If Action Subsystem2 : Subsystem  TreatAsAtomicUnit=on
  If Action Subsystem3 : Subsystem  TreatAsAtomicUnit=on
  If Action Subsystem4 : Subsystem  TreatAsAtomicUnit=on
  If Action Subsystem5 : Subsystem  TreatAsAtomicUnit=on
  If Action Subsystem6 : Subsystem  TreatAsAtomicUnit=on
  If Action Subsystem7 : Subsystem  TreatAsAtomicUnit=on
  If Action Subsystem8 : Subsystem  TreatAsAtomicUnit=on
  If Action Subsystem9 : Subsystem  TreatAsAtomicUnit=on
  If1 : If  NumInputs=2  IfExpression=(u1==15|u2==15)  ElseIfExpressions=(u1==6&u2==6),(u1==6&u2==10),(u1==6&u2==12)
  Merge : Merge  Inputs=5  InitialOutput=0
  Merge1 : Merge  Inputs=5  InitialOutput=0
  Out1 : Outport
  Out2 : Outport  Port=2
  wires:
  If Action Subsystem6/1(Out1) -> Merge/5
  Merge1/1 -> Out1/1
  If1/3 -> If Action Subsystem8/Action
  If1/2 -> If Action Subsystem5/Action
  If/2 -> If Action Subsystem1/Action
  If1/4 -> If Action Subsystem7/Action
  Merge/1 -> Out2/1
  <AEBSve_d_functionFARCState_convert>/1 -> If/1, If Action Subsystem6/1(In1)
  If Action Subsystem2/1(Out1) -> Merge/4
  <JABSve_d_DbFunFARCSta_convert>/1 -> If/2
  If Action Subsystem/1(Out1) -> Merge/1
  If Action Subsystem3/1(Out1) -> Merge/3
  If Action Subsystem7/1(Out1) -> Merge1/4
  If1/5 -> If Action Subsystem9/Action
  If/1 -> If Action Subsystem/Action
  If/3 -> If Action Subsystem3/Action
  If Action Subsystem5/1(Out1) -> Merge1/2
  <AEBSve_d_FCWStatus_convert>/1 -> If1/1, If Action Subsystem9/1(In1)
  If Action Subsystem4/1(Out1) -> Merge1/1
  If1/1 -> If Action Subsystem4/Action
  If Action Subsystem8/1(Out1) -> Merge1/3
  If Action Subsystem1/1(Out1) -> Merge/2
  If/5 -> If Action Subsystem6/Action
  If/4 -> If Action Subsystem2/Action
  If Action Subsystem9/1(Out1) -> Merge1/5
  <JABSve_d_DbJACWStatus_convert>/1 -> If1/2

== system OMAP/Runnable_OMAP_10ms_sys/OMAP_Module/Subsystem/IC_Arbitration/LKA_arb_ELK/Subsystem/Subsystem1 ==
  LKA_State : Inport
  ELK_State : Inport  Port=2
  AND{,1..3} (4 alike) : Logic  AllPortsSameDT=off  OutDataTypeStr=boolean
  Compare To Constant{,2,4,6} (4 alike) : simulink/Logic and Bit Operations/Compare To Constant  relop===  const=uint8(4)  OutDataTypeStr=boolean
  Compare To Constant{1,3,5,7} (4 alike) : simulink/Logic and Bit Operations/Compare To Constant  relop=~=  const=uint8(4)  OutDataTypeStr=boolean
  Unit Delay : UnitDelay  InitialCondition=uint8(0)  SampleTime=-1
  Unit Delay1 : UnitDelay  InitialCondition=uint8(0)  SampleTime=-1
  LKA_Up : Outport
  LKA_Down : Outport  Port=2
  LKA_Active : Outport  Port=3
  ELK_Up : Outport  Port=4
  ELK_Down : Outport  Port=5
  ELK_Active : Outport  Port=6
  wires:
  LKA_State/1 -> Compare To Constant/1, Unit Delay/1, Compare To Constant3/1
  Unit Delay/1 -> Compare To Constant2/1, Compare To Constant1/1
  Compare To Constant1/1 -> AND/1
  Compare To Constant/1 -> LKA_Active/1, AND/2
  AND/1 -> LKA_Up/1  "LKA_Up"
  Compare To Constant2/1 -> AND1/1
  Compare To Constant3/1 -> AND1/2
  AND1/1 -> LKA_Down/1  "LKA_Down"
  Compare To Constant4/1 -> ELK_Active/1, AND2/2
  Compare To Constant6/1 -> AND3/1
  AND3/1 -> ELK_Down/1  "ELK_Down"
  Compare To Constant5/1 -> AND2/1
  ELK_State/1 -> Compare To Constant4/1, Unit Delay1/1, Compare To Constant7/1
  Unit Delay1/1 -> Compare To Constant6/1, Compare To Constant5/1
  AND2/1 -> ELK_Up/1  "ELK_Up"
  Compare To Constant7/1 -> AND3/2

== system OMAP/Runnable_OMAP_10ms_sys/OMAP_Module/ICA_Direct_G59/ICA_Define/Subsystem1/Dspl/DsplPrcs/Icon ==
  note: 0：灭
      | 1：灰
      | 2：绿
      | 3：橙
      | 4：红
  note: 显示0条件：多车道模式选择ICA；
      | 显示1条件（灰色）：多车道模式选择TCL或ALC，THState~=0；
      | 显示2条件（绿色，不带AUTO）：多车道模式选择TLC，速度大于变道允许门槛值，THState=3；
      | 显示3条件（绿色，带AUTO）：多车道模式选择ALC，速度大于变道允许门槛值，THState=3；
      | 显示4条件（橙色）：多车道模式选择TLC或者ALC，速度大于变道允许门槛值，THState=4
      | 显示5条件（红色）：多车道模式选择TLC或者ALC，速度大于变道允许门槛值，THState=5
      | 之所以把速度条件加进来，其实是考虑到多车道功能的激活隐含了速度要大于某一门槛值这个条件
  note: 0：Default Value
      | 1：HWA Unavailable（未启用）
      | 2：HWA_TLC（触发式变道）
      | 3：HWA_ALC（主动变道）
      | 4：HWA_SL_SRR_Fail（硬件故障-功能无法开启或降级）
      | 5：HWA_Error（系统故障）
      | 6：Reserved（保留）
  note: 0 ：可以从降级回到正常，
      | 1 ：不可以从降级回到正常
  note: ACC_State【0：初始化；1：关闭；2：禁止；3：等待；4：激活；5：Override；6：只能制动；7：Cancel键退出；8：OFF键退出；15：故障】
  Icon_stTHState : Inport
  Icon_stACCState : Inport  Port=2
  Icon_dDgrdIconWarnHiDurnum : Inport  Port=3
  Icon_dDgrdIconWarnLoDurnum : Inport  Port=4
  Icon_dDgrdIconWarnflag : Inport  Port=5
  Icon_stTLC_ALCmodeSW : Inport  Port=6
  Icon_stLC_SpdCndtFlg : Inport  Port=7
  Bus Creator : BusCreator  Inputs=2
  Constant : Constant  Value=OMAP_ICA_iconSTATE0  OutDataTypeStr=uint16
  Constant1 : Constant  Value=OMAP_ICA_iconSTATE1  OutDataTypeStr=uint16
  Constant10 : Constant  Value=5  OutDataTypeStr=uint16
  Constant11 : Constant  OutDataTypeStr=uint16
  Constant12 : Constant  Value=0  OutDataTypeStr=uint16
  Constant13 : Constant  Value=OMAP_ICA_iconSTATE6  OutDataTypeStr=uint16
  Constant14 : Constant  Value=OMAP_ICA_iconSTATE7  OutDataTypeStr=uint16
  Constant15 : Constant  Value=OMAP_ICA_iconSTATE8  OutDataTypeStr=uint16
  Constant16 : Constant  Value=OMAP_ICA_iconSTATE4  OutDataTypeStr=uint16
  Constant2 : Constant  Value=OMAP_ICA_iconSTATE2  OutDataTypeStr=uint16
  Constant3 : Constant  Value=OMAP_ICA_iconSTATE3  OutDataTypeStr=uint16
  Constant4 : Constant  Value=OMAP_ICA_iconSTATE4  OutDataTypeStr=uint16
  Constant5 : Constant  Value=OMAP_ICA_iconSTATE5  OutDataTypeStr=uint16
  Constant6 : Constant  OutDataTypeStr=boolean
  Constant7 : Constant  Value=2  OutDataTypeStr=uint16
  Constant8 : Constant  Value=3  OutDataTypeStr=uint16
  Constant9 : Constant  Value=4  OutDataTypeStr=uint16
  If : If  NumInputs=2  IfExpression=u1==0  ElseIfExpressions=u1==1,u1==2,u1==3,u1==4,u1==5,u1==6,u1==7,(u1==8)&(u2~=4&u2~=5&u2~=6),(u1==8)&(u2==4|u2==5|u2==6)
  If Action Subsystem : Subsystem  TreatAsAtomicUnit=on
  If Action Subsystem1 : Subsystem  TreatAsAtomicUnit=on
  If Action Subsystem10 : Subsystem  TreatAsAtomicUnit=on
  If Action Subsystem11 : Subsystem  TreatAsAtomicUnit=on
  If Action Subsystem12 : Subsystem  TreatAsAtomicUnit=on
  If Action Subsystem13 : Subsystem  TreatAsAtomicUnit=on
  If Action Subsystem14 : Subsystem  TreatAsAtomicUnit=on
  If Action Subsystem15 : Subsystem  TreatAsAtomicUnit=on
  If Action Subsystem16 : Subsystem  TreatAsAtomicUnit=on
  If Action Subsystem2 : Subsystem  TreatAsAtomicUnit=on
  If Action Subsystem3 : Subsystem  TreatAsAtomicUnit=on
  If Action Subsystem4 : Subsystem  TreatAsAtomicUnit=on
  If Action Subsystem5 : Subsystem  TreatAsAtomicUnit=on
  If Action Subsystem6 : Subsystem  TreatAsAtomicUnit=on
  If Action Subsystem7 : Subsystem  TreatAsAtomicUnit=on
  If Action Subsystem8 : Subsystem  TreatAsAtomicUnit=on
  If Action Subsystem9 : Subsystem  TreatAsAtomicUnit=on
  If1 : If  IfExpression=u1 == 0
  If2 : If  NumInputs=3  IfExpression=u1==3&u2==2&u3==1  ElseIfExpressions=u1==3&u2==3&u3==1,u1==4&(u2==2|u2==3)&u3==1,u1==5&(u2==2|u2==3)&u3==1,u1~=0&(u2==2|u2==3)
  Merge : Merge  Inputs=11
  Merge1 : Merge
  Merge2 : Merge  Inputs=6
  Terminator : Terminator
  Terminator1 : Terminator
  Terminator2 : Terminator
  Unit Delay1 : UnitDelay  SampleTime=-1
  else : Subsystem  TreatAsAtomicUnit=on
  if : Subsystem  TreatAsAtomicUnit=on
  Icon_stIconDspl : Outport
  wires:
  Icon_stTHState/1 -> If2/1, If/1
  Icon_stACCState/1 -> If/2
  If/4 -> If Action Subsystem9/Action
  If/2 -> If Action Subsystem7/Action
  If/1 -> If Action Subsystem6/Action
  If/11 -> If Action Subsystem15/Action
  If/3 -> If Action Subsystem8/Action
  If/5 -> If Action Subsystem10/Action
  If Action Subsystem9/1(Out1) -> Merge/4
  Merge/1 -> Bus Creator/1, Unit Delay1/1  "Icon_stICAIcon"
  Unit Delay1/1 -> If Action Subsystem12/1(In1), If Action Subsystem15/1(In1), If Action Subsystem13/1(In1)
  If Action Subsystem6/1(Out1) -> Merge/1
  If Action Subsystem7/1(Out1) -> Merge/2
  If Action Subsystem8/1(Out1) -> Merge/3
  If Action Subsystem10/1(Out1) -> Merge/5
  If Action Subsystem11/1(Out1) -> Merge/6
  Constant/1 -> If Action Subsystem6/1(In1)
  Constant4/1 -> If Action Subsystem10/1(In1)
  Constant1/1 -> If Action Subsystem7/1(In1)
  Constant2/1 -> If Action Subsystem8/1(In1)
  If1/1 -> if/Action
  If1/2 -> else/Action
  Constant6/1 -> if/1(In1)
  if/1(Out1) -> Merge1/1
  Merge1/1 -> Terminator/1  "orange_enable"
  else/2(counter_status) -> Merge1/2
  Icon_dDgrdIconWarnflag/1 -> If1/1  "DgrdIconWarnflag"
  Icon_dDgrdIconWarnHiDurnum/1 -> else/1(HiDurnum)  "DgrdIconWarnHinum"
  Icon_dDgrdIconWarnLoDurnum/1 -> else/2(LoDurnum)  "DgrdIconWarnLonum"
  Icon_stTLC_ALCmodeSW/1 -> If2/2  "DgrdIconWarnLonum"
  Icon_stLC_SpdCndtFlg/1 -> If2/3  "DgrdIconWarnLonum"
  If2/1 -> If Action Subsystem/Action
  Constant7/1 -> If Action Subsystem/1(In1)
  If Action Subsystem/1(Out1) -> Merge2/1
  Constant8/1 -> If Action Subsystem1/1(In1)
  If2/2 -> If Action Subsystem1/Action
  If Action Subsystem1/1(Out1) -> Merge2/2
  Constant9/1 -> If Action Subsystem2/1(In1)
  If2/3 -> If Action Subsystem2/Action
  If Action Subsystem2/1(Out1) -> Merge2/3
  Constant10/1 -> If Action Subsystem3/1(In1)
  If2/4 -> If Action Subsystem3/Action
  If Action Subsystem3/1(Out1) -> Merge2/4
  Constant11/1 -> If Action Subsystem4/1(In1)
  If2/5 -> If Action Subsystem4/Action
  If Action Subsystem4/1(Out1) -> Merge2/5
  Constant12/1 -> If Action Subsystem5/1(In1)
  If2/6 -> If Action Subsystem5/Action
  If Action Subsystem5/1(Out1) -> Merge2/6
  Merge2/1 -> Bus Creator/2  "Icon_stHWAmode"
  Bus Creator/1 -> Icon_stIconDspl/1
  Constant3/1 -> If Action Subsystem9/1(In1)
  Constant5/1 -> If Action Subsystem11/1(In1)
  If/6 -> If Action Subsystem11/Action
  If/7 -> If Action Subsystem12/Action
  If Action Subsystem12/1(Out1) -> Merge/7
  If/8 -> If Action Subsystem13/Action
  If Action Subsystem13/1(Out1) -> Merge/8
  Constant15/1 -> If Action Subsystem14/1(In1)
  If/9 -> If Action Subsystem14/Action
  If Action Subsystem14/1(Out1) -> Merge/9
  If Action Subsystem15/1(Out1) -> Merge/11
  Constant13/1 -> Terminator1/1
  Constant14/1 -> Terminator2/1
  Constant16/1 -> If Action Subsystem16/1(In1)
  If/10 -> If Action Subsystem16/Action
  If Action Subsystem16/1(Out1) -> Merge/10
